simulink model "Obsv"  (R2023a)
settings: Solver=VariableStepAuto  StartTime=0.0  StopTime=100  RelTol=1e-3
values from neighbouring files (symbols this model uses):
  AL = A-L*C    [Script_Dirigibile.m]
  BL = [B L]    [Script_Dirigibile.m]
  C = C(1,:)    [Script_Dirigibile.m]
  ueq = u_eq    [Script_Dirigibile.m]
  x0_tilde = [x0(1)-xeq(1) x0(2)-xeq(2) x0(3)-xeq(3)]    [Script_Dirigibile.m]
  yeq = x_eq    [Script_Dirigibile.m]
undefined symbols (not defined in the file or in its folder): A, B
settings Model: Creator=giuco  LastModifiedBy=giuco

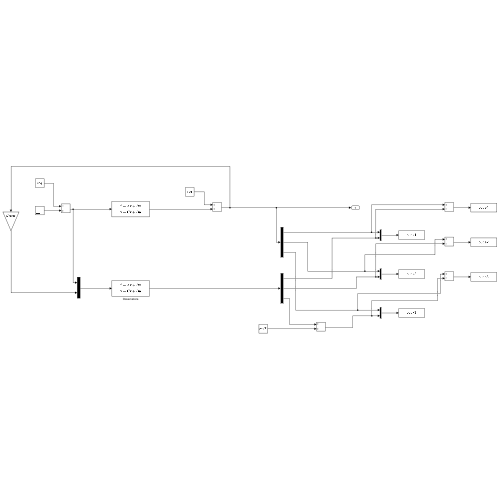
[thumbnail: Simulink's stored preview of the top-level diagram]
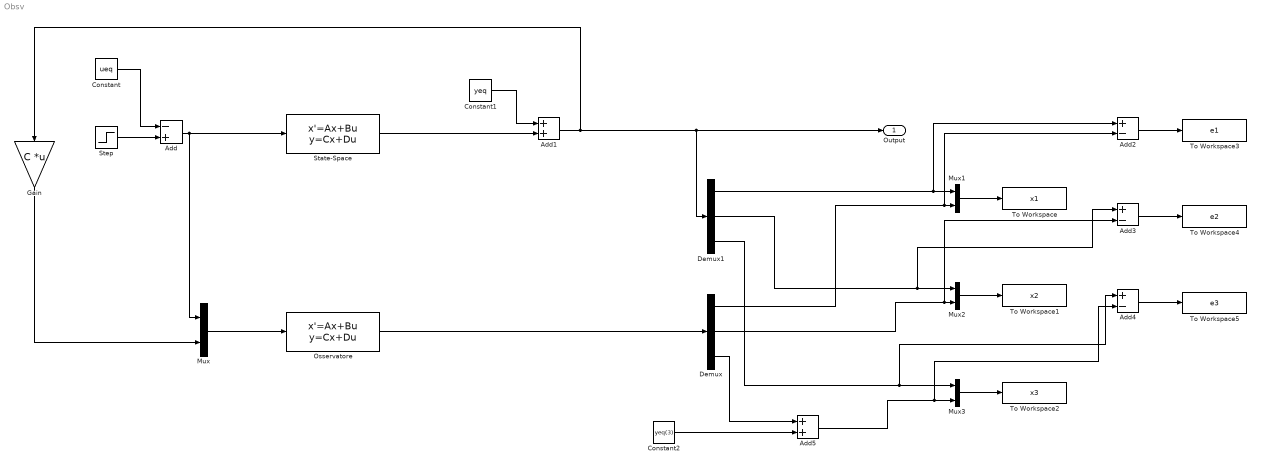
== system Obsv ==
  Add : Sum  Inputs=-+
  Add1 : Sum
  Add2 : Sum  Inputs=+-
  Add3 : Sum  Inputs=+-
  Add4 : Sum  Inputs=+-
  Add5 : Sum
  Constant : Constant  Value=ueq
  Constant1 : Constant  Value=yeq
  Constant2 : Constant  Value=yeq(3)
  Demux : Demux  Outputs=3
  Demux1 : Demux  Outputs=3
  Gain : Gain  Gain=C  Multiplication=Matrix(K*u) (u vector)
  Mux{,1..3} (4 alike) : Mux  Inputs=2
  Osservatore : StateSpace  A=AL  B=BL  C=eye(3)  D=zeros(3,2)  InitialCondition=[ 0 0 0 ]'
  State-Space : StateSpace  A=A  B=B  C=eye(3)  D=zeros(3,1)  InitialCondition=x0_tilde
  Step : Step  Time=0  After=1500  SampleTime=0
  To Workspace : ToWorkspace  VariableName=x1  SaveFormat=Timeseries  SampleTime=-1
  To Workspace1 : ToWorkspace  VariableName=x2  SaveFormat=Timeseries  SampleTime=-1
  To Workspace2 : ToWorkspace  VariableName=x3  SaveFormat=Timeseries  SampleTime=-1
  To Workspace3 : ToWorkspace  VariableName=e1  SaveFormat=Timeseries  SampleTime=-1
  To Workspace4 : ToWorkspace  VariableName=e2  SaveFormat=Timeseries  SampleTime=-1
  To Workspace5 : ToWorkspace  VariableName=e3  SaveFormat=Timeseries  SampleTime=-1
  Output : Outport
  wires:
  Step/1 -> Add/2
  Constant/1 -> Add/1
  Add/1 -> Mux/1, State-Space/1
  State-Space/1 -> Add1/2
  Constant1/1 -> Add1/1
  Add1/1 -> Gain/1, Demux1/1, Output/1
  Mux/1 -> Osservatore/1
  Demux1/1 -> Mux1/1, Add2/1
  Demux/1 -> Add2/2, Mux1/2
  Mux1/1 -> To Workspace/1
  Mux2/1 -> To Workspace1/1
  Demux1/2 -> Mux2/1, Add3/1
  Demux/2 -> Add3/2, Mux2/2
  Mux3/1 -> To Workspace2/1
  Demux1/3 -> Mux3/1, Add4/1
  Gain/1 -> Mux/2
  Add2/1 -> To Workspace3/1
  Add3/1 -> To Workspace4/1
  Add4/1 -> To Workspace5/1
  Osservatore/1 -> Demux/1
  Demux/3 -> Add5/1
  Constant2/1 -> Add5/2
  Add5/1 -> Add4/2, Mux3/2
